simulink model "MAGNETOMETER"  (R2024b)
settings: Solver=ode8  StartTime=0.0  StopTime=10000.0  FixedStep=0.02  RelTol=1e-3
undefined symbols (not defined in the file or in its folder): flag, sens
settings Model: Creator=parrot  LastModifiedBy=esteb

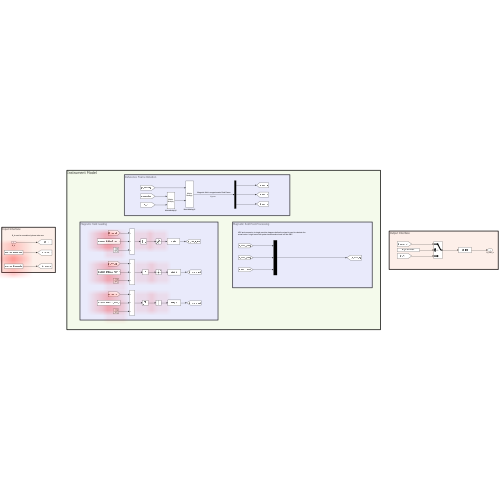
[thumbnail: Simulink's stored preview of the top-level diagram]
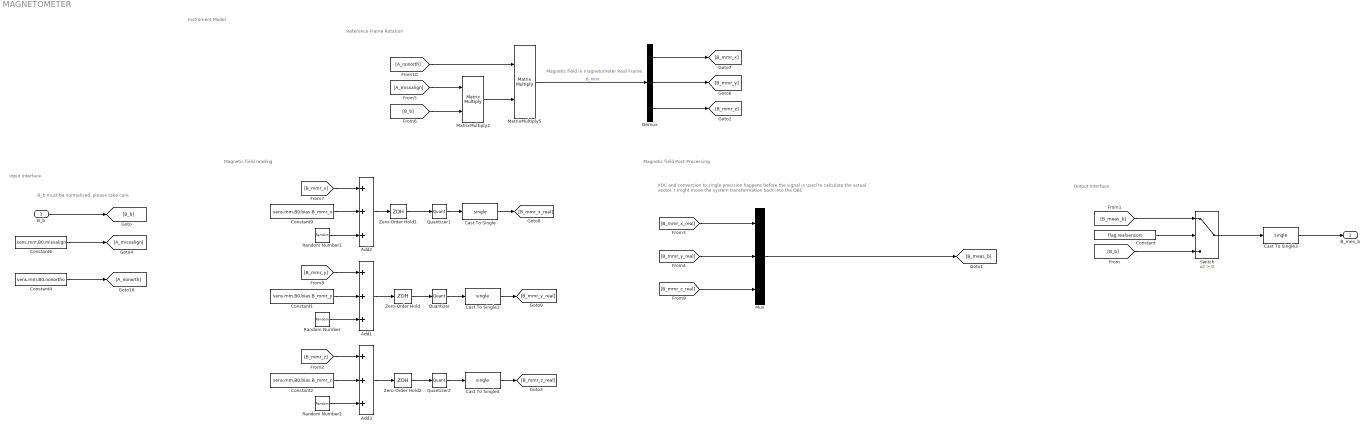
== system MAGNETOMETER ==
  note: Input Interface
  note: Reference Frame Rotation
  note: Instrument Model
  note: B_b must be normalised, please take care
  note: ADC and conversion to single precision happens before the signal is used to calculate the actual vector. I might move the system transformation back into the OBC
  note: Magnetic field Post-Processing
  note: Magnetic field reading
  note: Output Interface
  note: Magnetic field in magnetometer Real Frame
  B_b : Inport
  Add1 : Sum  Inputs=+++
  Add2 : Sum  Inputs=+++
  Add3 : Sum  Inputs=+++
  Cast To Single{,1,3..4} (4 alike) : DataTypeConversion  OutDataTypeStr=single  SaturateOnIntegerOverflow=off  RndMeth=Floor
  Constant : Constant  Value=flag.realsensors
  Constant1 : Constant  Value=sens.mm.B0.bias.B_mmr_y
  Constant2 : Constant  Value=sens.mm.B0.bias.B_mmr_z
  Constant4 : Constant  Value=sens.mm.B0.nonortho
  Constant6 : Constant  Value=sens.mm.B0.missalign
  Constant9 : Constant  Value=sens.mm.B0.bias.B_mmr_x
  Demux : Demux  Outputs=3
  MatrixMultiply2 : Product  Multiplication=Matrix(*)
  MatrixMultiply5 : Product  Multiplication=Matrix(*)
  Mux : Mux  Inputs=3
  Quantizer : Quantizer  QuantizationInterval=sens.mm.ADC.quanta
  Quantizer1 : Quantizer  QuantizationInterval=sens.mm.ADC.quanta
  Quantizer2 : Quantizer  QuantizationInterval=sens.mm.ADC.quanta
  Random Number : RandomNumber  Variance=(sens.mm.precision/1.4)^2  Seed=sens.mm.B0.seed.B_mmr_y  SampleTime=sens.mm.freq
  Random Number1 : RandomNumber  Variance=(sens.mm.precision/1.4)^2  Seed=sens.mm.B0.seed.B_mmr_x  SampleTime=sens.mm.freq
  Random Number2 : RandomNumber  Variance=(sens.mm.precision/1.4)^2  Seed=sens.mm.B0.seed.B_mmr_z  SampleTime=sens.mm.freq
  Switch : Switch  Criteria=u2 > Threshold  SaturateOnIntegerOverflow=off  InputSameDT=off
  Zero-Order Hold : ZeroOrderHold  SampleTime=sens.mm.freq
  Zero-Order Hold1 : ZeroOrderHold  SampleTime=sens.mm.freq
  Zero-Order Hold2 : ZeroOrderHold  SampleTime=sens.mm.freq
  B_mes_b : Outport
  wires:
  [B_mmr_y_real] -> Mux/2
  [B_mmr_z_real] -> Mux/3
  Add3/1 -> Zero-Order Hold2/1
  Zero-Order Hold2/1 -> Quantizer2/1
  Demux/1 -> [B_mmr_x]
  MatrixMultiply5/1 -> Demux/1  "B_mmr"
  Switch/1 -> Cast To Single3/1
  [B_mmr_z] -> Add3/1
  [B_mmr_x_real] -> Mux/1
  Demux/3 -> [B_mmr_z]
  [A_nonorth] -> MatrixMultiply5/1
  MatrixMultiply2/1 -> MatrixMultiply5/2
  Constant4/1 -> [A_nonorth]
  Constant6/1 -> [A_missalign]
  Random Number2/1 -> Add3/3
  [A_missalign] -> MatrixMultiply2/1
  Zero-Order Hold/1 -> Quantizer/1
  Demux/2 -> [B_mmr_y]
  Cast To Single3/1 -> B_mes_b/1
  [B_mmr_x] -> Add2/1
  Zero-Order Hold1/1 -> Quantizer1/1
  Add1/1 -> Zero-Order Hold/1
  [B_b] -> MatrixMultiply2/2
  [B_mmr_y] -> Add1/1
  Constant/1 -> Switch/2
  Cast To Single1/1 -> [B_mmr_y_real]
  Add2/1 -> Zero-Order Hold1/1
  Constant2/1 -> Add3/2
  Constant9/1 -> Add2/2
  Random Number1/1 -> Add2/3
  Quantizer1/1 -> Cast To Single/1
  Constant1/1 -> Add1/2
  Quantizer/1 -> Cast To Single1/1
  Cast To Single4/1 -> [B_mmr_z_real]
  B_b/1 -> [B_b]
  Mux/1 -> [B_meas_b]
  [B_b] -> Switch/3
  [B_meas_b] -> Switch/1
  Cast To Single/1 -> [B_mmr_x_real]
  Random Number/1 -> Add1/3
  Quantizer2/1 -> Cast To Single4/1
